simulink model "untitled"  (R2014a)
settings: Solver=ode45  StartTime=0.0  StopTime=10.0  RelTol=1e-3
libraries: neural x25
(part 1 of 4)
settings Model: Creator=CQU  LastModifiedBy=CQU

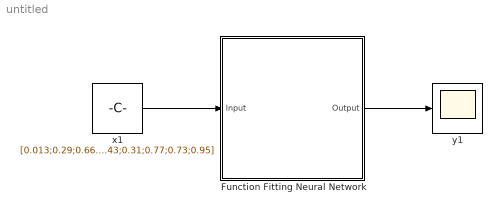
== system untitled ==
  Function Fitting Neural Network : Subsystem
      mask help: Function Fitting Neural Network
      mask Display: e = 0.06;c1 = [120 150 230]/255;c2 = ([120 150 230]+0)/383;c3 = ([120 150 230]+128)/383;patch([0 1 1 0],[0 0 1 1],c1);patch([0 1 1 1-e 1-e 0+e],[0 0 1 1-e 0+e 0+e],c2);patch([0 0 1 1-e 0+e 0+e],[0 1 1 1-e 1-e 0+e],c3);plot([0 1 1 0 0],[0 0 1 1 0]);fprintf('NNET');port_label('input',1,' Input');port_label('output',1,'Output ');
  x1 : Constant  Value=[0.013;0.29;0.66;0.51;0.13;0.017;0.059;0.32;0.027;0.71;0.12;0.027;0.36;0.6;0.98;0.58;0.12;0.29;0.27;0.23;0.083;0.25;0.68;0.99;0.51;0.036;0.07;0.22;0.29;0.74;0.96;0.0058;0.074;0.67;0.41;0.75;0.75;0.56;0.72;0.25;0.89;0.59;0.3;0.45;0.95;0.19;0.61;0.35;0.45;0.68;0.48;0.2;0.11;0.1;0.32;0.28;0.82;0.9;0.72;0.1;0.5;0.2;0.1;0.73;0.037;0.15;0.82;0.053;0.63;0.99;0.96;0.79;0.068;0.69;0.84;0.67;0.64;0.86;0.48;0.22;0.91;0.88;0.94;0.71;0.85;0.74;0.46;0.72;0.21;0.067;0.72;0.78;0.32;0.83;0.28;0.97;0.55;0.39;0.18;0.62;0.77;0.19;0.093;0.91;0.83;0.96;0.59;0.32;0.3;0.87;0.17;0.7;0.93;0.5;0.67;0.14;0.71;0.46;0.48;0.29;0.049;0.9;0.16;0.72;0.94;0.74;0.9;0.24;0.93;0.43;0.16;0.38;0.56;0.96;0.089;0.41;0.86;0.35;0.57;0.92;0.85;0.39;0.31;0.012;0.8;0.59;0.64;0.39;0.98;0.95;0.16;0.42;0.68;0.48;0.88;0.31;0.88;0.034;0.64;0.66;0.97;0.2;0.89;0.41;0.66;0.11;0.97;0.072;0.24;0.9;0.9;0.3;0.39;0.86;0.73;0.43;0.011;0.54;0.37;0.25;0.42;0.13;0.58;0.72;0.2;0.81;0.31;0.16;0.21;0.51;0.7;0.7;0.39;0.11;0.005;0.045;0.69;0.63;0.86;0.93;0.96;0.32;0.86;0.8;0.18;0.36;0.11;0.52;0.1;0.074;0.033;0.19;0.16;0.24;0.13;0.59;0.85;0.53;0.46;0.0083;0.055;0.55;0.89;0.68;0.57;0.95;0.46;0.58;0.98;0.44;0.85;0.93;0.72;0.44;0.46;0.49;0.3;0.16;0.61;0.075;0.9;0.87;0.044;0.7;0.72;0.56;0.7;0.035;0.27;0.12;0.69;0.91;0.87;0.36;0.016;0.052;0.84;0.52;0.024;0.09;0.43;0.22;0.36;0.58;0.61;0.28;0.89;0.11;0.69;0.41;0.39;0.73;0.56;0.38;0.64;0.62;0.32;0.54;0.72;0.36;0.83;0.24;0.43;0.76;0.21;0.33;0.6;0.47;0.47;0.29;0.65;0.98;0.76;0.43;0.75;0.46;0.45;0.83;0.33;0.22;0.19;0.11;0.64;0.53;0.59;0.64;0.64;0.6;0.44;0.59;0.61;0.063;0.37;0.98;0.11;0.77;0.46;0.072;0.68;0.33;0.38;0.15;0.88;0.54;0.7;0.25;0.67;0.67;0.41;0.64;0.74;0.26;0.029;0.53;0.38;0.79;0.47;0.61;0.16;0.6;0.19;0.15;0.86;0.99;0.29;0.39;0.37;0.94;0.7;0.12;0.36;0.28;0.14;0.39;0.21;0.43;0.65;0.89;0.76;0.66;0.28;0.57;0.84;0.94;0.39;0.6;0.26;0.65;0.24;0.087;0.31;0.51;0.98;0.042;0.075;0.77;0.47;0.91;0.99;0.08;0.064;0.32;0.41;0.35;0.47;0.4;0.79;0.39;0.77;0.33;0.95;0.24;0.85;0.11;0.15;0.4;0.65;0.73;0.7;0.45;0.62;0.55;0.35;0.81;0.087;0.16;0.019;0.22;0.41;0.73;0.82;0.88;0.1;0.95;0.78;0.5;0.024;0.59;0.85;0.67;0.89;0.38;0.093;0.88;0.59;0.84;0.52;0.52;0.72;0.56;0.04;0.58;0.21;0.94;0.02;0.94;0.31;0.58;0.96;0.11;0.6;0.73;0.67;0.36;0.11;0.022;0.92;0.69;0.78;0.23;0.69;0.11;0.014;0.63;0.79;0.68;0.3;0.54;0.94;0.065;0.44;0.34;0.87;0.058;0.75;0.51;0.45;0.33;0.19;0.98;0.089;0.28;0.46;0.66;0.39;0.76;0.84;0.95;0.086;0.26;0.63;0.43;0.4;0.37;0.2;0.93;0.57;0.26;0.66;0.18;0.98;0.7;0.13;0.13;0.37;0.85;0.14;0.54;0.95;0.26;0.093;0.013;0.81;0.34;0.47;0.21;0.22;0.58;0.34;0.32;0.83;0.61;0.19;0.97;0.78;0.14;0.97;0.69;0.94;0.16;0.023;0.11;0.22;0.3;0.21;0.97;0.78;0.13;0.15;0.4;0.39;0.12;0.64;0.87;0.33;0.44;0.74;0.36;0.024;0.11;0.043;0.29;0.27;0.75;0.9;0.33;0.94;0.94;0.45;0.28;0.17;0.063;0.31;0.23;0.45;0.18;0.1;0.95;0.53;0.43;0.22;0.78;0.49;0.56;0.99;0.9;0.7;0.32;0.51;0.98;0.11;0.42;0.94;0.92;0.48;0.66;0.25;0.39;0.48;0.7;0.35;0.45;0.42;0.056;0.68;0.79;0.44;0.63;0.54;0.4;0.24;0.61;0.61;0.84;0.72;0.27;0.21;0.027;0.36;0.43;0.46;0.12;0.4;0.41;0.75;0.9;0.53;0.36;0.52;0.36;0.89;0.24;0.093;0.99;0.66;0.44;0.89;0.32;0.29;0.54;0.97;0.55;0.46;0.99;0.95;0.98;0.79;0.72;0.54;0.39;0.36;0.18;0.52;0.69;0.76;0.091;0.97;0.34;0.22;0.52;0.6;0.34;0.91;0.86;0.63;0.89;0.23;0.43;0.62;0.41;0.98;0.79;0.64;0.98;0.59;0.77;0.25;0.017;0.47;0.12;0.48;0.62;0.91;0.94;0.23;0.072;0.52;0.48;0.94;0.1;0.12;0.34;0.11;0.19;0.81;0.14;0.84;0.43;0.74;0.79;0.97;0.93;0.39;0.79;0.00096;0.74;0.01;0.51;0.91;0.36;0.13;0.56;0.65;0.59;0.67;0.44;0.21;0.49;0.31;0.94;0.13;0.78;0.07;0.75;0.54;0.32;0.54;0.66;0.48;0.99;0.59;0.33;0.46;0.97;0.49;0.9;0.14;0.99;0.87;0.75;0.43;0.47;0.67;1;0.64;0.46;0.73;0.89;0.61;0.66;0.21;0.082;0.28;0.23;0.95;0.065;0.36;0.57;0.19;0.033;0.22;0.23;1;0.27;0.028;0.42;0.081;0.18;0.81;0.04;0.66;0.63;0.15;0.53;0.013;0.48;0.27;0.86;0.59;0.21;0.47;0.61;0.22;0.51;0.97;0.55;0.46;0.33;0.86;0.3;0.83;0.92;0.2;0.28;0.62;0.93;0.98;1;0.51;0.41;0.51;0.41;0.51;0.81;0.32;0.33;0.61;0.98;0.79;0.17;0.45;0.13;0.65;0.04;0.096;0.025;0.72;0.47 ...(+20049 chars)]  SampleTime=1
      mask Display: e = 0.06;c1 = [120 230 180]/255;c2 = ([120 230 180]+0)/(256+128);c3 = ([120 230 180]+128)/(256+128);patch([0 1 1 0],[0 0 1 1],c1);patch([0 1 1 1-e 1-e 0+e],[0 0 1 1-e 0+e 0+e],c2);patch([0 0 1 1-e 0+e 0+e],[0 1 1 1-e 1-e 0+e],c3);plot([0 1 1 0 0],[0 0 1 1 0]);disp('Constant');
  y1 : Scope
      mask Display: e = 0.06;c1 = [120 230 180]/255;c2 = ([120 230 180]+0)/(256+128);c3 = ([120 230 180]+128)/(256+128);patch([0 1 1 0],[0 0 1 1],c1);patch([0 1 1 1-e 1-e 0+e],[0 0 1 1-e 0+e 0+e],c2);patch([0 0 1 1-e 0+e 0+e],[0 1 1 1-e 1-e 0+e],c3);plot([0 1 1 0 0],[0 0 1 1 0]);plot([0.15 0.85 0.85 0.15 0.15],[0.5 0.5 0.85 0.85 0.5]);
  wires:
  x1/1 -> Function Fitting Neural Network/1(Input)
  Function Fitting Neural Network/1(Output) -> y1/1

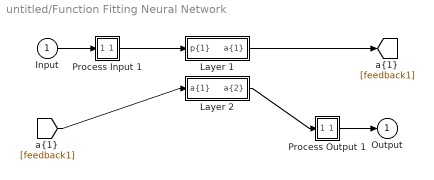
== system untitled/Function Fitting Neural Network ==
  Input : Inport  PortDimensions=4800
      mask Display: e = 0.06;c1 = [120 230 180]/255;c2 = ([120 230 180]+0)/(256+128);c3 = ([120 230 180]+128)/(256+128);patch([0 1 1 0],[0 0 1 1],c1);patch([0 1 1 1-e 1-e 0+e],[0 0 1 1-e 0+e 0+e],c2);patch([0 0 1 1-e 0+e 0+e],[0 1 1 1-e 1-e 0+e],c3);plot([0 1 1 0 0],[0 0 1 1 0]);
  Layer 1 : Subsystem
      mask Display: e = 0.06;c1 = [120 150 230]/255;c2 = ([120 150 230]+0)/383;c3 = ([120 150 230]+128)/383;patch([0 1 1 0],[0 0 1 1],c1);patch([0 1 1 1-e 1-e 0+e],[0 0 1 1-e 0+e 0+e],c2);patch([0 0 1 1-e 0+e 0+e],[0 1 1 1-e 1-e 0+e],c3);plot([0 1 1 0 0],[0 0 1 1 0]);
  Layer 2 : Subsystem
      mask Display: e = 0.06;c1 = [120 150 230]/255;c2 = ([120 150 230]+0)/383;c3 = ([120 150 230]+128)/383;patch([0 1 1 0],[0 0 1 1],c1);patch([0 1 1 1-e 1-e 0+e],[0 0 1 1-e 0+e 0+e],c2);patch([0 0 1 1-e 0+e 0+e],[0 1 1 1-e 1-e 0+e],c3);plot([0 1 1 0 0],[0 0 1 1 0]);
  Process Input 1 : Subsystem
      mask Display: e = 0.06;c1 = [120 150 230]/255;c2 = ([120 150 230]+0)/383;c3 = ([120 150 230]+128)/383;patch([0 1 1 0],[0 0 1 1],c1);patch([0 1 1 1-e 1-e 0+e],[0 0 1 1-e 0+e 0+e],c2);patch([0 0 1 1-e 0+e 0+e],[0 1 1 1-e 1-e 0+e],c3);plot([0 1 1 0 0],[0 0 1 1 0]);
  Process Output 1 : Subsystem
      mask Display: e = 0.06;c1 = [120 150 230]/255;c2 = ([120 150 230]+0)/383;c3 = ([120 150 230]+128)/383;patch([0 1 1 0],[0 0 1 1],c1);patch([0 1 1 1-e 1-e 0+e],[0 0 1 1-e 0+e 0+e],c2);patch([0 0 1 1-e 0+e 0+e],[0 1 1 1-e 1-e 0+e],c3);plot([0 1 1 0 0],[0 0 1 1 0]);
  Output : Outport  InitialOutput=0
      mask Display: e = 0.06;c1 = [120 230 180]/255;c2 = ([120 230 180]+0)/(256+128);c3 = ([120 230 180]+128)/(256+128);patch([0 1 1 0],[0 0 1 1],c1);patch([0 1 1 1-e 1-e 0+e],[0 0 1 1-e 0+e 0+e],c2);patch([0 0 1 1-e 0+e 0+e],[0 1 1 1-e 1-e 0+e],c3);plot([0 1 1 0 0],[0 0 1 1 0]);
  wires:
  Input/1 -> Process Input 1/1(x)
  Process Output 1/1(y) -> Output/1
  Process Input 1/1(p) -> Layer 1/1("p{1}")
  Layer 1/1("a{1}") -> [feedback1]
  [feedback1] -> Layer 2/1("a{1} ")
  Layer 2/1("a{2}") -> Process Output 1/1(a)

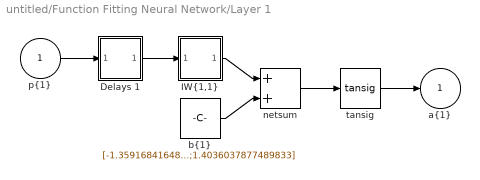
== system untitled/Function Fitting Neural Network/Layer 1 ==
  "p{1}" : Inport  PortDimensions=4800
      mask Display: e = 0.06;c1 = [120 230 180]/255;c2 = ([120 230 180]+0)/(256+128);c3 = ([120 230 180]+128)/(256+128);patch([0 1 1 0],[0 0 1 1],c1);patch([0 1 1 1-e 1-e 0+e],[0 0 1 1-e 0+e 0+e],c2);patch([0 0 1 1-e 0+e 0+e],[0 1 1 1-e 1-e 0+e],c3);plot([0 1 1 0 0],[0 0 1 1 0]);
  Delays 1 : Subsystem
      mask Display: e = 0.06;c1 = [120 150 230]/255;c2 = ([120 150 230]+0)/383;c3 = ([120 150 230]+128)/383;patch([0 1 1 0],[0 0 1 1],c1);patch([0 1 1 1-e 1-e 0+e],[0 0 1 1-e 0+e 0+e],c2);patch([0 0 1 1-e 0+e 0+e],[0 1 1 1-e 1-e 0+e],c3);plot([0 1 1 0 0],[0 0 1 1 0]);disp('0');
  "IW{1,1}" : Subsystem
      mask Display: e = 0.06;c1 = [120 150 230]/255;c2 = ([120 150 230]+0)/383;c3 = ([120 150 230]+128)/383;patch([0 1 1 0],[0 0 1 1],c1);patch([0 1 1 1-e 1-e 0+e],[0 0 1 1-e 0+e 0+e],c2);patch([0 0 1 1-e 0+e 0+e],[0 1 1 1-e 1-e 0+e],c3);plot([0 1 1 0 0],[0 0 1 1 0]);disp('W');
  "b{1}" : Constant  Value=[-1.3591684164839462;-1.2542492424012608;-1.104713726743473;-0.96143366612327241;0.81436875504268502;0.64322161520346355;-0.5252815710149028;0.35242783784621406;-0.2027214551539227;-0.073357531065857656;0.087228351435731571;-0.20357976677146611;-0.3545411962357497;0.52218200725293451;-0.6756570708659394;-0.81271596137742075;-0.94210093124104544;-1.1087481576922331;1.257169579856279;1.4036037877489833]
      mask Display: e = 0.06;c1 = [120 150 230]/255;c2 = ([120 150 230]+0)/383;c3 = ([120 150 230]+128)/383;patch([0 1 1 0],[0 0 1 1],c1);patch([0 1 1 1-e 1-e 0+e],[0 0 1 1-e 0+e 0+e],c2);patch([0 0 1 1-e 0+e 0+e],[0 1 1 1-e 1-e 0+e],c3);plot([0 1 1 0 0],[0 0 1 1 0]);disp('b');
  netsum : Sum  Inputs=2  SaturateOnIntegerOverflow=on  InputSameDT=on  OutDataTypeStr=Inherit: Same as first input
      mask Display: e = 0.06;c1 = [120 150 230]/255;c2 = ([120 150 230]+0)/383;c3 = ([120 150 230]+128)/383;patch([0 1 1 0],[0 0 1 1],c1);patch([0 1 1 1-e 1-e 0+e],[0 0 1 1-e 0+e 0+e],c2);patch([0 0 1 1-e 0+e 0+e],[0 1 1 1-e 1-e 0+e],c3);plot([0 1 1 0 0],[0 0 1 1 0]);disp('+');
  tansig : neural/Transfer Functions/tansig
  "a{1}" : Outport  InitialOutput=[0;0;0;0;0;0;0;0;0;0;0;0;0;0;0;0;0;0;0;0]
      mask Display: e = 0.06;c1 = [120 230 180]/255;c2 = ([120 230 180]+0)/(256+128);c3 = ([120 230 180]+128)/(256+128);patch([0 1 1 0],[0 0 1 1],c1);patch([0 1 1 1-e 1-e 0+e],[0 0 1 1-e 0+e 0+e],c2);patch([0 0 1 1-e 0+e 0+e],[0 1 1 1-e 1-e 0+e],c3);plot([0 1 1 0 0],[0 0 1 1 0]);
  wires:
  "p{1}"/1 -> Delays 1/1("p{1}")
  Delays 1/1("pd{1,1}") -> "IW{1,1}"/1("pd{1,1}")
  "IW{1,1}"/1("iz{1,1}") -> netsum/1
  "b{1}"/1 -> netsum/2
  netsum/1 -> tansig/1
  tansig/1 -> "a{1}"/1

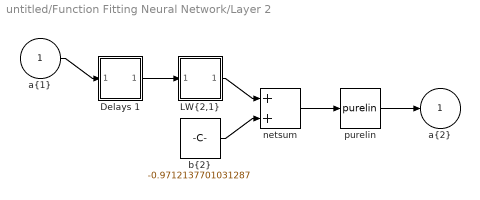
== system untitled/Function Fitting Neural Network/Layer 2 ==
  "a{1} " : Inport  PortDimensions=20
      mask Display: e = 0.06;c1 = [120 230 180]/255;c2 = ([120 230 180]+0)/(256+128);c3 = ([120 230 180]+128)/(256+128);patch([0 1 1 0],[0 0 1 1],c1);patch([0 1 1 1-e 1-e 0+e],[0 0 1 1-e 0+e 0+e],c2);patch([0 0 1 1-e 0+e 0+e],[0 1 1 1-e 1-e 0+e],c3);plot([0 1 1 0 0],[0 0 1 1 0]);
  Delays 1 : Subsystem
      mask Display: e = 0.06;c1 = [120 150 230]/255;c2 = ([120 150 230]+0)/383;c3 = ([120 150 230]+128)/383;patch([0 1 1 0],[0 0 1 1],c1);patch([0 1 1 1-e 1-e 0+e],[0 0 1 1-e 0+e 0+e],c2);patch([0 0 1 1-e 0+e 0+e],[0 1 1 1-e 1-e 0+e],c3);plot([0 1 1 0 0],[0 0 1 1 0]);disp('0');
  "LW{2,1}" : Subsystem
      mask Display: e = 0.06;c1 = [120 150 230]/255;c2 = ([120 150 230]+0)/383;c3 = ([120 150 230]+128)/383;patch([0 1 1 0],[0 0 1 1],c1);patch([0 1 1 1-e 1-e 0+e],[0 0 1 1-e 0+e 0+e],c2);patch([0 0 1 1-e 0+e 0+e],[0 1 1 1-e 1-e 0+e],c3);plot([0 1 1 0 0],[0 0 1 1 0]);disp('W');
  "b{2}" : Constant  Value=-0.9712137701031287
      mask Display: e = 0.06;c1 = [120 150 230]/255;c2 = ([120 150 230]+0)/383;c3 = ([120 150 230]+128)/383;patch([0 1 1 0],[0 0 1 1],c1);patch([0 1 1 1-e 1-e 0+e],[0 0 1 1-e 0+e 0+e],c2);patch([0 0 1 1-e 0+e 0+e],[0 1 1 1-e 1-e 0+e],c3);plot([0 1 1 0 0],[0 0 1 1 0]);disp('b');
  netsum : Sum  Inputs=2  SaturateOnIntegerOverflow=on  InputSameDT=on  OutDataTypeStr=Inherit: Same as first input
      mask Display: e = 0.06;c1 = [120 150 230]/255;c2 = ([120 150 230]+0)/383;c3 = ([120 150 230]+128)/383;patch([0 1 1 0],[0 0 1 1],c1);patch([0 1 1 1-e 1-e 0+e],[0 0 1 1-e 0+e 0+e],c2);patch([0 0 1 1-e 0+e 0+e],[0 1 1 1-e 1-e 0+e],c3);plot([0 1 1 0 0],[0 0 1 1 0]);disp('+');
  purelin : neural/Transfer Functions/purelin
  "a{2}" : Outport  InitialOutput=0
      mask Display: e = 0.06;c1 = [120 230 180]/255;c2 = ([120 230 180]+0)/(256+128);c3 = ([120 230 180]+128)/(256+128);patch([0 1 1 0],[0 0 1 1],c1);patch([0 1 1 1-e 1-e 0+e],[0 0 1 1-e 0+e 0+e],c2);patch([0 0 1 1-e 0+e 0+e],[0 1 1 1-e 1-e 0+e],c3);plot([0 1 1 0 0],[0 0 1 1 0]);
  wires:
  "a{1} "/1 -> Delays 1/1("p{2}")
  Delays 1/1("pd{2,1}") -> "LW{2,1}"/1("ad{2,1}")
  "LW{2,1}"/1("lz{2,1}") -> netsum/1
  "b{2}"/1 -> netsum/2
  netsum/1 -> purelin/1
  purelin/1 -> "a{2}"/1
